simulink model "pmsm_l"  (R2022b)
settings: Solver=VariableStepAuto  StartTime=0.0  StopTime=simParam.stopTime  MaxStep=simParam.maxStep  RelTol=1e-3
values from neighbouring files (symbols this model uses):
  linear =     [linearSystem.mat]
undefined symbols (not defined in the file or in its folder): aug
settings Model: Creator=KAIQUE-GCA  LastModifiedBy=kaike

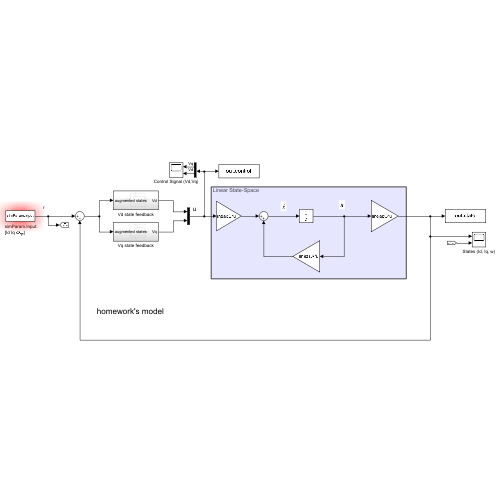
[thumbnail: Simulink's stored preview of the top-level diagram]
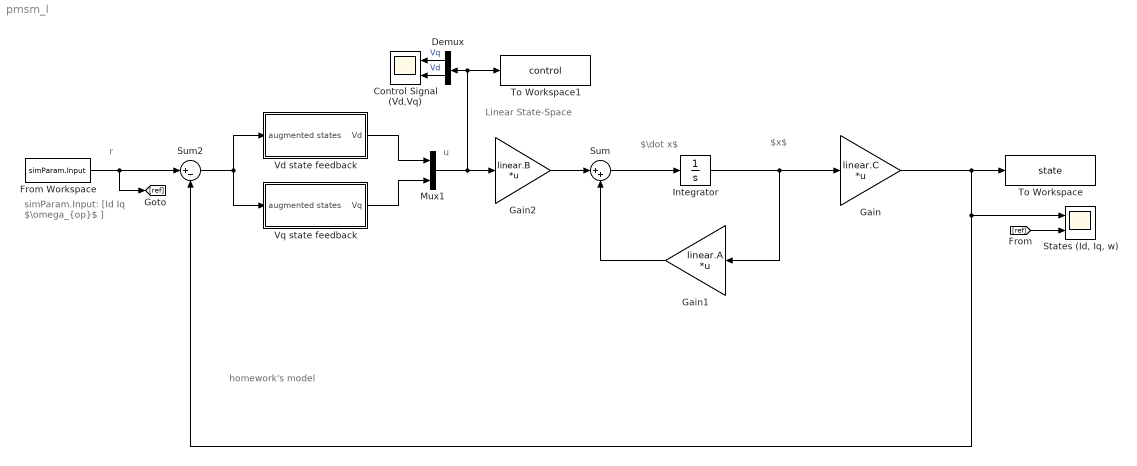
== system pmsm_l ==
  note: r
  note: simParam.Input:
      | [Id Iq $\omega_{op}$ ]
  note: u
  note: Linear State-Space
  note: homework's model
  note: $x$
  note: $\dot x$
  Control Signal (Vd,Vq) : Scope  NumInputPorts=2
  Demux : Demux  Outputs=2
  From Workspace : FromWorkspace  VariableName=simParam.Input  OutputAfterFinalValue=Holding final value
  Gain : Gain  Gain=linear.C  Multiplication=Matrix(K*u)
  Gain1 : Gain  Gain=linear.A  Multiplication=Matrix(K*u)
  Gain2 : Gain  Gain=linear.B  Multiplication=Matrix(K*u)
  Integrator : Integrator
  Mux1 : Mux  Inputs=2
  "States (Id, Iq, w)" : Scope  NumInputPorts=2
  Sum : Sum  Inputs=|++
  Sum2 : Sum  Inputs=|+-
  To Workspace : ToWorkspace  VariableName=state  SampleTime=-1
  To Workspace1 : ToWorkspace  VariableName=control  SampleTime=-1
  Vd state feedback : Subsystem
  Vq state feedback : Subsystem
  wires:
  Gain2/1 -> Sum/1
  Integrator/1 -> Gain1/1, Gain/1
  Gain/1 -> To Workspace/1, Sum2/2, "States (Id, Iq, w)"/1
  Gain1/1 -> Sum/2
  Sum/1 -> Integrator/1
  Mux1/1 -> To Workspace1/1, Demux/1, Gain2/1
  Vq state feedback/1(Vq) -> Mux1/2
  Vd state feedback/1(Vd) -> Mux1/1
  Sum2/1 -> Vq state feedback/1(augmented states), Vd state feedback/1(augmented states)
  From Workspace/1 -> Sum2/1, [ref]
  [ref] -> "States (Id, Iq, w)"/2
  Demux/1 -> Control Signal (Vd,Vq)/1  "Vq"
  Demux/2 -> Control Signal (Vd,Vq)/2  "Vd"

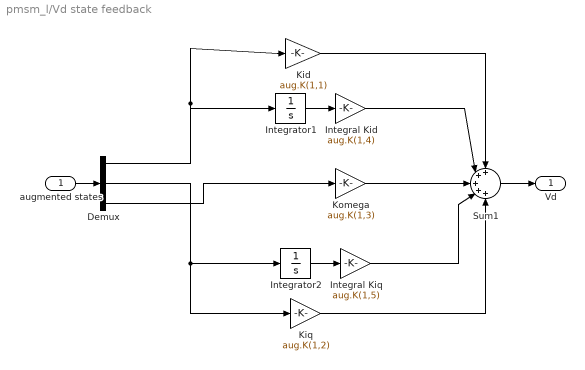
== system pmsm_l/Vd state feedback ==
  augmented states : Inport
  Demux : Demux  Outputs=3
  Integral Kid : Gain  Gain=aug.K(1,4)
  Integral Kiq : Gain  Gain=aug.K(1,5)
  Integrator1 : Integrator
  Integrator2 : Integrator
  Kid : Gain  Gain=aug.K(1,1)
  Kiq : Gain  Gain=aug.K(1,2)
  Komega : Gain  Gain=aug.K(1,3)
  Sum1 : Sum  Inputs=+++++
  Vd : Outport
  wires:
  augmented states/1 -> Demux/1
  Integrator1/1 -> Integral Kid/1
  Sum1/1 -> Vd/1
  Integrator2/1 -> Integral Kiq/1
  Demux/1 -> Kid/1, Integrator1/1
  Integral Kid/1 -> Sum1/2
  Kid/1 -> Sum1/1
  Demux/3 -> Komega/1
  Komega/1 -> Sum1/3
  Demux/2 -> Kiq/1, Integrator2/1
  Integral Kiq/1 -> Sum1/4
  Kiq/1 -> Sum1/5

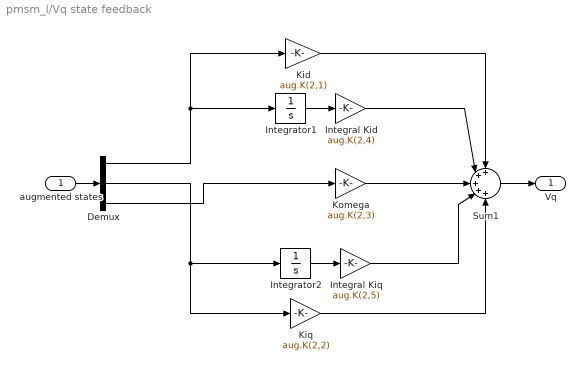
== system pmsm_l/Vq state feedback ==
  augmented states : Inport
  Demux : Demux  Outputs=3
  Integral Kid : Gain  Gain=aug.K(2,4)
  Integral Kiq : Gain  Gain=aug.K(2,5)
  Integrator1 : Integrator
  Integrator2 : Integrator
  Kid : Gain  Gain=aug.K(2,1)
  Kiq : Gain  Gain=aug.K(2,2)
  Komega : Gain  Gain=aug.K(2,3)
  Sum1 : Sum  Inputs=+++++
  Vq : Outport
  wires:
  augmented states/1 -> Demux/1
  Integrator1/1 -> Integral Kid/1
  Sum1/1 -> Vq/1
  Integrator2/1 -> Integral Kiq/1
  Demux/1 -> Kid/1, Integrator1/1
  Integral Kid/1 -> Sum1/2
  Kid/1 -> Sum1/1
  Demux/3 -> Komega/1
  Komega/1 -> Sum1/3
  Demux/2 -> Kiq/1, Integrator2/1
  Integral Kiq/1 -> Sum1/4
  Kiq/1 -> Sum1/5
